simulink model "SUMARSONO_Simulink_Hamming_Code"  (R2013a)
settings: Solver=ode45  SolverMode=SingleTasking  StartTime=0.0  StopTime=inf  RelTol=1e-3
undefined symbols (not defined in the file): gfprimfd
libraries: commblkcod2 x2, commrandsrc2 x1, commchan3 x1, commsink2 x1
settings Model: Creator=The MathWorks Inc.  LastModifiedBy=CQ42
settings DataIOCC: SignalLoggingSaveFormat=ModelDataLogs  SaveOutput=off  SaveTime=off  SignalLoggingName=sigsOut
settings OptimizationCC: BooleanDataType=off  InlineParams=on  ExpressionDepthLimit=2147483647
settings DebuggingCC: AlgebraicLoopMsg=error  SaveWithParameterizedLinksMsg=none  SignalResolutionControl=TryResolveAllWithWarning  SolverPrmCheckMsg=none  MultiTaskDSMMsg=warning  MultiTaskCondExecSysMsg=none  FcnCallInpInsideContextMsg=UseLocalSettings  StrictBusMsg=None
settings HardwareCC: TargetIntDivRoundTo=Zero  TargetEndianess=LittleEndian  TargetHWDeviceType=MATLAB Host  ProdEqTarget=off
settings RTWCC: IncludeERTFirstTime=on
settings GRTTargetCC: CombineOutputUpdateFcns=off  GRTInterface=on

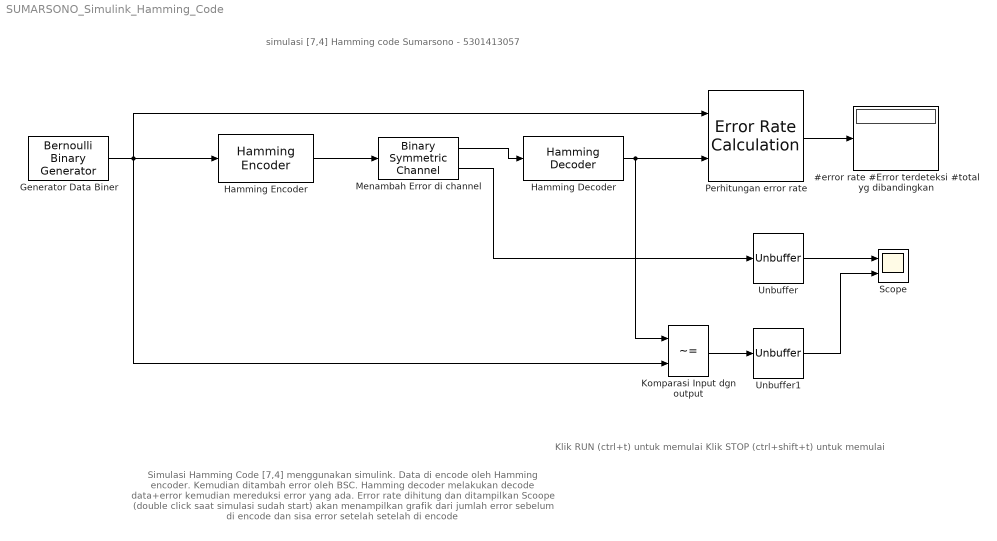
== system SUMARSONO_Simulink_Hamming_Code ==
  note: simulasi [7,4] Hamming code
      | Sumarsono - 5301413057
  note: Simulasi Hamming Code [7,4] menggunakan simulink.
      | Data di encode oleh Hamming encoder.
      | Kemudian ditambah error oleh BSC.
      | Hamming decoder melakukan decode data+error kemudian mereduksi error yang ada.
      | Error rate dihitung dan ditampilkan
      |
      | Scoope (double click saat simulasi sudah start) akan menampilkan grafik dari
      | jumlah error sebelum di encode
      | dan sisa error setelah setelah di encode
  note: Klik RUN (ctrl+t) untuk memulai
      | Klik STOP (ctrl+shift+t) untuk memulai
  " #error rate #Error terdeteksi #total yg dibandingkan " : Display
  Generator Data Biner : commrandsrc2/Bernoulli Binary Generator  P=0.5  seed=61  Ts=1  frameBased=on  sampPerFrame=4  orient=off  outDataType=double
  Hamming Decoder : commblkcod2/Hamming Decoder  n=7  k=gfprimfd(3,'min')
  Hamming Encoder : commblkcod2/Hamming Encoder  n=7  k=gfprimfd(3,'min')
  Komparasi Input dgn output : RelationalOperator  Operator=~=  OutDataTypeStr=boolean
  Menambah Error di channel : commchan3/Binary Symmetric Channel  P=0.01  s=2137  E=on  outDtype=double
  Perhitungan error rate : commsink2/Error Rate Calculation  N=0  st_delay=0  cp_mode=Entire frame  subframe=[]  PMode=Port  WsName=ErrorVec  RsMode2=off  stop=off  numErr=100  maxBits=1e6
  Scope : Scope  NumInputPorts=2
      settings: TimeRange=5000  YMin=-1~-1  YMax=2~2  MaxDataPoints=30000
  Unbuffer : Unbuffer  SampleBasedProcessing=Same as frame based
  Unbuffer1 : Unbuffer  SampleBasedProcessing=Same as frame based
  wires:
  Perhitungan error rate/1 -> " #error rate #Error terdeteksi #total yg dibandingkan "/1
  Generator Data Biner/1 -> Komparasi Input dgn output/2, Hamming Encoder/1, Perhitungan error rate/1
  Menambah Error di channel/1 -> Hamming Decoder/1
  Hamming Encoder/1 -> Menambah Error di channel/1
  Hamming Decoder/1 -> Komparasi Input dgn output/1, Perhitungan error rate/2
  Menambah Error di channel/2 -> Unbuffer/1
  Komparasi Input dgn output/1 -> Unbuffer1/1
  Unbuffer1/1 -> Scope/2
  Unbuffer/1 -> Scope/1
